simulink model "ForwardDynamics"  (Simulink 8.8)
settings: Solver=VariableStepAuto  StartTime=0.0  StopTime=4  FixedStep=0.01  MaxStep=0.08  RelTol=1e-3  EnableMultiTasking=on
settings Model: Creator=gwu  LastModifiedBy=Guilherme
settings OptimizationCC: ExpressionDepthLimit=2147483647
settings DebuggingCC: SolverPrmCheckMsg=warning
settings RTWCC: TargetLang=C++
settings GRTTargetCC: CombineOutputUpdateFcns=on  GRTInterface=off

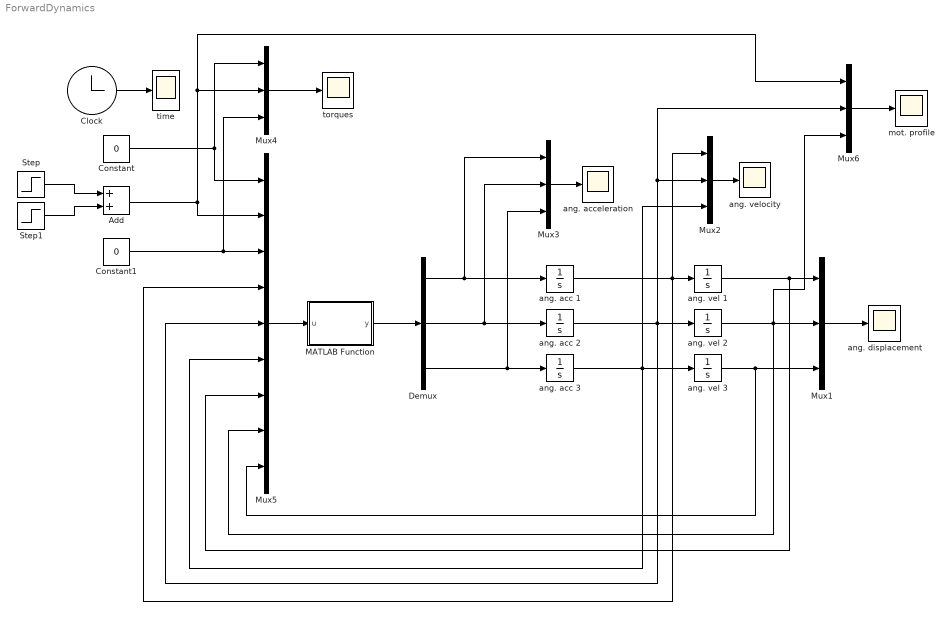
== system ForwardDynamics ==
  Add : Sum
  Clock : Clock
  Constant : Constant  Value=0
  Constant1 : Constant  Value=0
  Demux : Demux  Outputs=3
  MATLAB Function : MATLAB Function  TreatAsAtomicUnit=on
  Mux{1..4,6} (5 alike) : Mux  Inputs=3
  Mux5 : Mux  Inputs=9
  Step : Step  Time=0  SampleTime=0
  Step1 : Step  After=-1  SampleTime=0
  ang. acc 1 : Integrator
  ang. acc 2 : Integrator
  ang. acc 3 : Integrator
  ang. acceleration : Scope
  ang. displacement : Scope
  ang. vel 1 : Integrator
  ang. vel 2 : Integrator
  ang. vel 3 : Integrator
  ang. velocity : Scope
  mot. profile : Scope
  time : Scope
  torques : Scope
  wires:
  ang. acc 1/1 -> Mux5/4, ang. vel 1/1, Mux2/1
  ang. vel 1/1 -> Mux5/7, Mux1/1
  ang. vel 2/1 -> Mux6/3, Mux5/8, Mux1/2
  ang. acc 2/1 -> Mux5/5, ang. vel 2/1, Mux6/2, Mux2/2
  Demux/1 -> ang. acc 1/1, Mux3/1
  Demux/2 -> ang. acc 2/1, Mux3/2
  Mux1/1 -> ang. displacement/1
  Mux2/1 -> ang. velocity/1
  Mux3/1 -> ang. acceleration/1
  Clock/1 -> time/1
  Mux4/1 -> torques/1
  Demux/3 -> Mux3/3, ang. acc 3/1
  ang. acc 3/1 -> Mux5/6, Mux2/3, ang. vel 3/1
  ang. vel 3/1 -> Mux5/9, Mux1/3
  Step/1 -> Add/1
  Step1/1 -> Add/2
  Constant/1 -> Mux5/1, Mux4/1
  Mux5/1 -> MATLAB Function/1(u)
  MATLAB Function/1(y) -> Demux/1
  Mux6/1 -> mot. profile/1
  Add/1 -> Mux6/1, Mux4/2, Mux5/2
  Constant1/1 -> Mux4/3, Mux5/3

== matlab function MATLAB Function ==
  data: u input double size=9; y output double size=3
function y = fcn(u)

y = ForwardDyn_L2([u(1); u(2); u(3); u(4); u(5); u(6); u(7); u(8); u(9)]);
